simulink model "NMPC_PID"  (R2024a)
settings: Solver=FixedStepAuto  StartTime=0.0  StopTime=130  FixedStep=0.05  RelTol=1e-3
PostLoadFcn:
  | on_model_load
InitFcn:
  | on_model_start
StopFcn:
  | on_simulation_done
model workspace (MAT data in the model file):
  ActiveExperiment.Id = '85ae8ae8-3421-447e-86e6-f1860a57dbe5'
  ActiveExperiment.Name = "Two steps high noise"
  ActiveExperiment.Description = ""
  ActiveExperiment.ConstHorizonReference = 0
  ActiveExperiment.ComponentType = "scenario"
  ActiveExperiment.SimulationTime = 60
  ActiveExperiment.Subcomponents = "Disturbance"
  ActiveExperiment.Disturbance.Id = 'ccaeaedb-34fb-4469-93e3-0e771cb356d7'
  ActiveExperiment.Disturbance.Name = 'New Disturbance'
  ActiveExperiment.Disturbance.Description = ''
  ActiveExperiment.Disturbance.LibVersionHash = ''
  ActiveExperiment.Disturbance.Lib = 'csbenchlab'
  ActiveExperiment.Disturbance.LibVersion = '0.0.1'
  ActiveExperiment.Disturbance.PluginType = 'dist'
  ActiveExperiment.Disturbance.PluginName = 'Gauss'
  ActiveExperiment.Disturbance.PluginImplementation = 'mat'
  ActiveExperiment.Disturbance.ParentComponentId = '85ae8ae8-3421-447e-86e6-f1860a57dbe5'
  ActiveExperiment.Disturbance.ParentComponentType = 'scenario'
  ActiveExperiment.Disturbance.ComponentType = 'disturbance'
  ActiveExperiment.Disturbance.ParentComponentName = 'Two steps high noise'
  ActiveExperiment.SystemIc = [0; 0; 0; 0; 0; 0; 0; 0; 0; 0; 0; 0]
  ActiveExperiment.SystemParameterOverrides.payload_mass.timeseries__ = 1
  ActiveExperiment.SystemParameterOverrides.payload_mass.data = [0  0; 30  20]
  ActiveExperiment.SystemParameterOverrides.payload_location.timeseries__ = 1
  ActiveExperiment.SystemParameterOverrides.payload_location.data = [0 0 -0.15 0]
  ActiveExperiment.SystemParameterOverrides.current_speed = 0.2
  ActiveExperiment.SystemParameterOverrides.current_direction = 0.1
  ActiveExperiment.Reference = '/home/luka/fer/csbenchlab_gym/envs/marine_otter_full/data/references/85ae8ae8-3421-447e-86e6-f1860a57dbe5_ref.mat'
  ActiveExperiment.DisturbanceParameterOverrides = struct()
  ActiveExperiment.NumEvaluations = 1
  ActiveExperiment.RandomSeed = 42
  ActiveExperiment.SystemParams.payload_mass = timeseries
  ActiveExperiment.SystemParams.payload_mass.Name = 'unnamed'
  ActiveExperiment.SystemParams.payload_mass.DataInfo = tsdata.datametadata
  ActiveExperiment.SystemParams.payload_mass.DataInfo.Interpolation = tsdata.interpolation
  ActiveExperiment.SystemParams.payload_mass.DataInfo.Interpolation.Fhandle : function handle (value not decoded)
  ActiveExperiment.SystemParams.payload_mass.DataInfo.Interpolation.Name = 'linear'
  ActiveExperiment.SystemParams.payload_mass.TimeInfo = tsdata.timemetadata
  ActiveExperiment.SystemParams.payload_mass.TimeInfo.Length = 2
  ActiveExperiment.SystemParams.payload_mass.TimeInfo.DuplicateTimes = 0
  ActiveExperiment.SystemParams.payload_mass.TimeInfo.Time_ = [0; 30]
  ActiveExperiment.SystemParams.payload_mass.TimeInfo.Initialized = 1
  ActiveExperiment.SystemParams.payload_mass.QualityInfo = tsdata.qualmetadata
  ActiveExperiment.SystemParams.payload_mass.Data_ = [0; 20]
  ActiveExperiment.SystemParams.payload_location = timeseries
  ActiveExperiment.SystemParams.payload_location.Name = 'unnamed'
  ActiveExperiment.SystemParams.payload_location.DataInfo = tsdata.datametadata
  ActiveExperiment.SystemParams.payload_location.DataInfo.Interpolation = tsdata.interpolation
  ActiveExperiment.SystemParams.payload_location.DataInfo.Interpolation.Fhandle : function handle (value not decoded)
  ActiveExperiment.SystemParams.payload_location.DataInfo.Interpolation.Name = 'linear'
  ActiveExperiment.SystemParams.payload_location.TimeInfo = tsdata.timemetadata
  ActiveExperiment.SystemParams.payload_location.TimeInfo.Length = 1
  ActiveExperiment.SystemParams.payload_location.TimeInfo.DuplicateTimes = 0
  ActiveExperiment.SystemParams.payload_location.TimeInfo.Time_ = 0
  ActiveExperiment.SystemParams.payload_location.TimeInfo.Initialized = 1
  ActiveExperiment.SystemParams.payload_location.QualityInfo = tsdata.qualmetadata
  ActiveExperiment.SystemParams.payload_location.Data_ = [0 -0.15 0]
  ActiveExperiment.SystemParams.current_speed = timeseries
  ActiveExperiment.SystemParams.current_speed.Name = 'unnamed'
  ActiveExperiment.SystemParams.current_speed.DataInfo = tsdata.datametadata
  ActiveExperiment.SystemParams.current_speed.DataInfo.Interpolation = tsdata.interpolation
  ActiveExperiment.SystemParams.current_speed.DataInfo.Interpolation.Fhandle : function handle (value not decoded)
  ActiveExperiment.SystemParams.current_speed.DataInfo.Interpolation.Name = 'linear'
  ActiveExperiment.SystemParams.current_speed.TimeInfo = tsdata.timemetadata
  ActiveExperiment.SystemParams.current_speed.TimeInfo.Length = 1
  ActiveExperiment.SystemParams.current_speed.TimeInfo.DuplicateTimes = 0
  ActiveExperiment.SystemParams.current_speed.TimeInfo.Time_ = 0
  ActiveExperiment.SystemParams.current_speed.TimeInfo.Initialized = 1
  ActiveExperiment.SystemParams.current_speed.QualityInfo = tsdata.qualmetadata
  ActiveExperiment.SystemParams.current_speed.Data_ = 0.2
  ActiveExperiment.SystemParams.current_direction = timeseries
  ActiveExperiment.SystemParams.current_direction.Name = 'unnamed'
  ActiveExperiment.SystemParams.current_direction.DataInfo = tsdata.datametadata
  ActiveExperiment.SystemParams.current_direction.DataInfo.Interpolation = tsdata.interpolation
  ActiveExperiment.SystemParams.current_direction.DataInfo.Interpolation.Fhandle : function handle (value not decoded)
  ActiveExperiment.SystemParams.current_direction.DataInfo.Interpolation.Name = 'linear'
  ActiveExperiment.SystemParams.current_direction.TimeInfo = tsdata.timemetadata
  ActiveExperiment.SystemParams.current_direction.TimeInfo.Length = 1
  ActiveExperiment.SystemParams.current_direction.TimeInfo.DuplicateTimes = 0
  ActiveExperiment.SystemParams.current_direction.TimeInfo.Time_ = 0
  ActiveExperiment.SystemParams.current_direction.TimeInfo.Initialized = 1
  ActiveExperiment.SystemParams.current_direction.QualityInfo = tsdata.qualmetadata
  ActiveExperiment.SystemParams.current_direction.Data_ = 0.1
  ActiveExperiment.SystemParams.out_gain = timeseries
  ActiveExperiment.SystemParams.out_gain.Name = 'unnamed'
  ActiveExperiment.SystemParams.out_gain.DataInfo = tsdata.datametadata
  ActiveExperiment.SystemParams.out_gain.DataInfo.Interpolation = tsdata.interpolation
  ActiveExperiment.SystemParams.out_gain.DataInfo.Interpolation.Fhandle : function handle (value not decoded)
  ActiveExperiment.SystemParams.out_gain.DataInfo.Interpolation.Name = 'linear'
  ActiveExperiment.SystemParams.out_gain.TimeInfo = tsdata.timemetadata
  ActiveExperiment.SystemParams.out_gain.TimeInfo.Length = 1
  ActiveExperiment.SystemParams.out_gain.TimeInfo.DuplicateTimes = 0
  ActiveExperiment.SystemParams.out_gain.TimeInfo.Time_ = 0
  ActiveExperiment.SystemParams.out_gain.TimeInfo.Initialized = 1
  ActiveExperiment.SystemParams.out_gain.QualityInfo = tsdata.qualmetadata
  ActiveExperiment.SystemParams.out_gain.Data_ = 1
  Experiments(1).Id = '1e1e735a-ca72-47f3-9e23-ef054322de06'
  Experiments(1).Name = "Five steps perturbed high noise"
  Experiments(1).Description = ""
  Experiments(1).ConstHorizonReference = 0
  Experiments(1).ComponentType = "scenario"
  Experiments(1).SimulationTime = 60
  Experiments(1).Subcomponents = "Disturbance"
  Experiments(1).Disturbance.Id = 'd00b25fa-299c-4dde-a026-233da86bc131'
  Experiments(1).Disturbance.Name = ''
  Experiments(1).Disturbance.Description = ''
  Experiments(1).Disturbance.LibVersionHash = ''
  Experiments(1).Disturbance.Lib = 'csbenchlab'
  Experiments(1).Disturbance.LibVersion = '0.0.1'
  Experiments(1).Disturbance.PluginType = 'dist'
  Experiments(1).Disturbance.PluginName = 'Gauss'
  Experiments(1).Disturbance.PluginImplementation = 'mat'
  Experiments(1).Disturbance.ParentComponentId = '1e1e735a-ca72-47f3-9e23-ef054322de06'
  Experiments(1).Disturbance.ParentComponentName = 'Five steps perturbed high noise'
  Experiments(1).Disturbance.ParentComponentType = 'scenario'
  Experiments(1).Disturbance.ComponentType = 'disturbance'
  Experiments(1).Disturbance.DestinationPath = 'disturbances'
  Experiments(1).SystemIc = [0; 0; 0; 0; 0; 0; 0; 0; 0; 0; 0; 0]
  Experiments(1).SystemParameterOverrides.payload_mass.timeseries__ = 1
  Experiments(1).SystemParameterOverrides.payload_mass.data = [0  35; 27  35]
  Experiments(1).Reference = '/home/luka/fer/csbenchlab_gym/envs/marine_otter_full/data/references/1e1e735a-ca72-47f3-9e23-ef054322de06_ref.mat'
  Experiments(1).DisturbanceParameterOverrides = struct()
  Experiments(1).NumEvaluations = 1000
  Experiments(1).RandomSeed = 42
  Experiments(2).Id = '1e727098-795b-40af-9168-30502f01196e'
  Experiments(2).Name = "Two steps"
  Experiments(2).Description = ""
  Experiments(2).ConstHorizonReference = 0
  Experiments(2).ComponentType = "scenario"
  Experiments(2).SimulationTime = 60
  Experiments(2).Subcomponents = "Disturbance"
  Experiments(2).Disturbance = struct()
  Experiments(2).SystemIc = [0; 0; 0; 0; 0; 0; 0; 0; 0; 0; 0; 0]
  Experiments(2).SystemParameterOverrides.payload_mass.timeseries__ = 1
  Experiments(2).SystemParameterOverrides.payload_mass.data = [0  0; 27  0]
  Experiments(2).Reference = '/home/luka/fer/csbenchlab_gym/envs/marine_otter_full/data/references/1e727098-795b-40af-9168-30502f01196e_ref.mat'
  Experiments(2).DisturbanceParameterOverrides = struct()
  Experiments(2).NumEvaluations = 1
  Experiments(2).RandomSeed = 42
  Experiments(3).Id = '832a0fb6-0823-4b09-93b7-a1f8c841e784'
  Experiments(3).Name = "Sinuses"
  Experiments(3).Description = ""
  Experiments(3).ConstHorizonReference = 0
  Experiments(3).ComponentType = "scenario"
  Experiments(3).SimulationTime = 60
  Experiments(3).Subcomponents = "Disturbance"
  Experiments(3).Disturbance.Id = '6582568e-6a07-4ca1-973d-ce726013b9e5'
  Experiments(3).Disturbance.Name = ''
  Experiments(3).Disturbance.Description = ''
  Experiments(3).Disturbance.LibVersionHash = ''
  Experiments(3).Disturbance.Lib = 'csbenchlab'
  Experiments(3).Disturbance.LibVersion = '0.0.1'
  Experiments(3).Disturbance.PluginType = 'dist'
  Experiments(3).Disturbance.PluginName = 'Gauss'
  Experiments(3).Disturbance.PluginImplementation = 'mat'
  Experiments(3).Disturbance.ParentComponentId = '832a0fb6-0823-4b09-93b7-a1f8c841e784'
  Experiments(3).Disturbance.ParentComponentName = 'Sinuses'
  Experiments(3).Disturbance.ParentComponentType = 'scenario'
  Experiments(3).Disturbance.ComponentType = 'disturbance'
  Experiments(3).Disturbance.DestinationPath = 'disturbances'
  Experiments(3).SystemIc = [0; 0; 0; 0; 0; 0; 0; 0; 0; 0; 0; 0]
  Experiments(3).SystemParameterOverrides.payload_mass.timeseries__ = 1
  Experiments(3).SystemParameterOverrides.payload_mass.data = [0  35; 12  35]
  Experiments(3).Reference = '/home/luka/fer/csbenchlab_gym/envs/marine_otter_full/data/references/832a0fb6-0823-4b09-93b7-a1f8c841e784_ref.mat'
  Experiments(3).DisturbanceParameterOverrides = struct()
  Experiments(3).NumEvaluations = 1000
  Experiments(3).RandomSeed = 42
  Experiments(4).Id = '85ae8ae8-3421-447e-86e6-f1860a57dbe5'
  Experiments(4).Name = "Two steps high noise"
  Experiments(4).Description = ""
  Experiments(4).ConstHorizonReference = 0
  Experiments(4).ComponentType = "scenario"
  Experiments(4).SimulationTime = 60
  Experiments(4).Subcomponents = "Disturbance"
  Experiments(4).Disturbance.Id = 'ccaeaedb-34fb-4469-93e3-0e771cb356d7'
  Experiments(4).Disturbance.Name = 'New Disturbance'
  Experiments(4).Disturbance.Description = ''
  Experiments(4).Disturbance.LibVersionHash = ''
  Experiments(4).Disturbance.Lib = 'csbenchlab'
  Experiments(4).Disturbance.LibVersion = '0.0.1'
  Experiments(4).Disturbance.PluginType = 'dist'
  Experiments(4).Disturbance.PluginName = 'Gauss'
  Experiments(4).Disturbance.PluginImplementation = 'mat'
  Experiments(4).Disturbance.ParentComponentId = '85ae8ae8-3421-447e-86e6-f1860a57dbe5'
  Experiments(4).Disturbance.ParentComponentType = 'scenario'
  Experiments(4).Disturbance.ComponentType = 'disturbance'
  Experiments(4).Disturbance.ParentComponentName = 'Two steps high noise'
  Experiments(4).SystemIc = [0; 0; 0; 0; 0; 0; 0; 0; 0; 0; 0; 0]
  Experiments(4).SystemParameterOverrides.payload_mass.timeseries__ = 1
  Experiments(4).SystemParameterOverrides.payload_mass.data = [0  0; 30  20]
  Experiments(4).SystemParameterOverrides.payload_location.timeseries__ = 1
  Experiments(4).SystemParameterOverrides.payload_location.data = [0 0 -0.15 0]
  Experiments(4).SystemParameterOverrides.current_speed = 0.2
  Experiments(4).SystemParameterOverrides.current_direction = 0.1
  Experiments(4).Reference = '/home/luka/fer/csbenchlab_gym/envs/marine_otter_full/data/references/85ae8ae8-3421-447e-86e6-f1860a57dbe5_ref.mat'
  Experiments(4).DisturbanceParameterOverrides = struct()
  Experiments(4).NumEvaluations = 1
  Experiments(4).RandomSeed = 42
  Experiments(5).Id = '9caafca7-6b3d-4fd5-b43b-2d0badebda60'
  Experiments(5).Name = "Five steps perturbed"
  Experiments(5).Description = ""
  Experiments(5).ConstHorizonReference = 0
  Experiments(5).ComponentType = "scenario"
  Experiments(5).SimulationTime = 60
  Experiments(5).Subcomponents = "Disturbance"
  Experiments(5).Disturbance.Id = '941af73e-12e7-42cf-853d-f79bb40068e7'
  Experiments(5).Disturbance.Name = ''
  Experiments(5).Disturbance.Description = ''
  Experiments(5).Disturbance.LibVersionHash = ''
  Experiments(5).Disturbance.Lib = 'csbenchlab'
  Experiments(5).Disturbance.LibVersion = '0.0.1'
  Experiments(5).Disturbance.PluginType = 'dist'
  Experiments(5).Disturbance.PluginName = 'Gauss'
  Experiments(5).Disturbance.PluginImplementation = 'mat'
  Experiments(5).Disturbance.ParentComponentId = '9caafca7-6b3d-4fd5-b43b-2d0badebda60'
  Experiments(5).Disturbance.ParentComponentName = 'Five steps perturbed'
  Experiments(5).Disturbance.ParentComponentType = 'scenario'
  Experiments(5).Disturbance.ComponentType = 'disturbance'
  Experiments(5).Disturbance.DestinationPath = 'disturbances'
  Experiments(5).SystemIc = [0; 0; 0; 0; 0; 0; 0; 0; 0; 0; 0; 0]
  Experiments(5).SystemParameterOverrides.payload_mass.timeseries__ = 1
  Experiments(5).SystemParameterOverrides.payload_mass.data = [0  0; 27  0]
  Experiments(5).Reference = '/home/luka/fer/csbenchlab_gym/envs/marine_otter_full/data/references/9caafca7-6b3d-4fd5-b43b-2d0badebda60_ref.mat'
  Experiments(5).DisturbanceParameterOverrides = struct()
  Experiments(5).NumEvaluations = 1000
  Experiments(5).RandomSeed = 42
  Experiments(6).Id = 'd997722b-b22e-4a88-a68f-d421073cfd81'
  Experiments(6).Name = "Sinuses high noise"
  Experiments(6).Description = ""
  Experiments(6).ConstHorizonReference = 0
  Experiments(6).ComponentType = "scenario"
  Experiments(6).SimulationTime = 60
  Experiments(6).Subcomponents = "Disturbance"
  Experiments(6).Disturbance.Id = 'e3fab669-38a8-480e-9185-300544970487'
  Experiments(6).Disturbance.Name = ''
  Experiments(6).Disturbance.Description = ''
  Experiments(6).Disturbance.LibVersionHash = ''
  Experiments(6).Disturbance.Lib = 'csbenchlab'
  Experiments(6).Disturbance.LibVersion = '0.0.1'
  Experiments(6).Disturbance.PluginType = 'dist'
  Experiments(6).Disturbance.PluginName = 'Gauss'
  Experiments(6).Disturbance.PluginImplementation = 'mat'
  Experiments(6).Disturbance.ParentComponentId = 'd997722b-b22e-4a88-a68f-d421073cfd81'
  Experiments(6).Disturbance.ParentComponentName = 'Sinuses high noise'
  Experiments(6).Disturbance.ParentComponentType = 'scenario'
  Experiments(6).Disturbance.ComponentType = 'disturbance'
  Experiments(6).Disturbance.DestinationPath = 'disturbances'
  Experiments(6).SystemIc = [0; 0; 0; 0; 0; 0; 0; 0; 0; 0; 0; 0]
  Experiments(6).SystemParameterOverrides.payload_mass.timeseries__ = 1
  Experiments(6).SystemParameterOverrides.payload_mass.data = [0  35; 12  35]
  Experiments(6).Reference = '/home/luka/fer/csbenchlab_gym/envs/marine_otter_full/data/references/d997722b-b22e-4a88-a68f-d421073cfd81_ref.mat'
  Experiments(6).DisturbanceParameterOverrides = struct()
  Experiments(6).NumEvaluations = 1000
  Experiments(6).RandomSeed = 42
  GlobalReference = 0
  callbacks = dictionary
  callbacks.data.Version = 1
  callbacks.data.IsKeyCombined = 1
  callbacks.data.IsValueCombined = 1
  callbacks.data.Key = ["on_start:31b52d05-ccc9-4eab-bb0e-3c80b4e6f477"; "on_start:f41ef9e4-ba34-416c-84b6-7794956a3c04"; "on_start:9c40ba40-a30c-4d47-b6ea-332d53085db4"; "on_start:a6a9c6d3-ff58-4f5d-b7b7-6a5809d04cef"; "on_start:59d3b695-31bd-4d38-a8d0-9c2b61ca3ebd"; "on_start:68187f7d-81f5-4756-96be-de0d65363a63"; "on_start:17c1b7c7-d1b2-4e6c-bab6-21ffb9ee4dcb"; "on_start:a5c8738f-8d38-4797-a21a-203fc6d46076"; "on_load:4a0d1010-4549-4d51-b3a5-602e7c932b45"; "on_start:4a0d1010-4549-4d51-b3a5-602e7c932b45"; "on_end:4a0d1010-4549-4d51-b3a5-602e7c932b45"]
  callbacks.data.Value{1}.external_function__ = 1
  callbacks.data.Value{1}.function = 'configure_controller_params'
  callbacks.data.Value{1}.backend = 'm'
  callbacks.data.Value{1}.kwargs = struct()
  callbacks.data.Value{2}.external_function__ = 1
  callbacks.data.Value{2}.function = 'configure_controller_params'
  callbacks.data.Value{2}.backend = 'm'
  callbacks.data.Value{2}.kwargs = struct()
  callbacks.data.Value{3}.external_function__ = 1
  callbacks.data.Value{3}.function = 'configure_controller_params'
  callbacks.data.Value{3}.backend = 'm'
  callbacks.data.Value{3}.kwargs = struct()
  callbacks.data.Value{4}.external_function__ = 1
  callbacks.data.Value{4}.function = 'configure_controller_params'
  callbacks.data.Value{4}.backend = 'm'
  callbacks.data.Value{4}.kwargs = struct()
  callbacks.data.Value{5}.external_function__ = 1
  callbacks.data.Value{5}.function = 'configure_controller_params'
  callbacks.data.Value{5}.backend = 'm'
  callbacks.data.Value{5}.kwargs = struct()
  callbacks.data.Value{6}.external_function__ = 1
  callbacks.data.Value{6}.function = 'configure_controller_params'
  callbacks.data.Value{6}.backend = 'm'
  callbacks.data.Value{6}.kwargs = struct()
  callbacks.data.Value{7}.external_function__ = 1
  callbacks.data.Value{7}.function = 'configure_controller_params'
  callbacks.data.Value{7}.backend = 'm'
  callbacks.data.Value{7}.kwargs = struct()
  callbacks.data.Value{8}.external_function__ = 1
  callbacks.data.Value{8}.function = 'configure_controller_params'
  callbacks.data.Value{8}.backend = 'm'
  callbacks.data.Value{8}.kwargs = struct()
  callbacks.data.Value{9} = py.function
  callbacks.data.Value{10} = py.function
  callbacks.data.Value{11} = py.function
  env_name = 'NMPC_PID'
  extrinsic = 1
  gen_blocks.systems.systems.Name = 'CS System'
  gen_blocks.systems.systems.Handle = 'NMPC_PID/CS System'
  gen_blocks.systems.systems.Path = 'NMPC_PID/CS System'
  gen_blocks.systems.systems.Disturbance = []
  gen_blocks.systems.systems.Id = "4a0d1010-4549-4d51-b3a5-602e7c932b45"
  gen_blocks.systems.systems.Components.Name = 'Otter'
  gen_blocks.systems.systems.Components.Handle = 1179.08288574
  gen_blocks.systems.systems.Components.Path = 'NMPC_PID/CS System/Otter'
  gen_blocks.systems.systems.Components.Id = "4a0d1010-4549-4d51-b3a5-602e7c932b45"
  gen_blocks.systems.systems.Components.LibPath = "marine_lib_sys/Otter"
  gen_blocks.systems.systems.SignalSubsystem = []
  gen_blocks.systems.dims.Inputs = 2
  gen_blocks.systems.dims.Outputs = 12
  gen_blocks.controllers.Name = 'CS Controller'
  gen_blocks.controllers.Handle = 'NMPC_PID/CS Controller'
  gen_blocks.controllers.Path = 'NMPC_PID/CS Controller'
  gen_blocks.controllers.Id = "8582e3e1-de85-466e-b412-44a269ccd2bf"
  gen_blocks.controllers.Components.Name = 'PID'
  gen_blocks.controllers.Components.Handle = 7921.01660156
  gen_blocks.controllers.Components.Path = 'NMPC_PID/CS Controller/PID'
  gen_blocks.controllers.Components.Id = "8582e3e1-de85-466e-b412-44a269ccd2bf"
  gen_blocks.controllers.Components.LibPath = "csbenchlab_ctl/PID"
  gen_blocks.controllers.Components.RefExtractor.Path = 'NMPC_PID/CS Controller/ref_extractor_1'
  gen_blocks.controllers.IoHandles.inport_y.h = 1033.08984375
  gen_blocks.controllers.IoHandles.inport_y.p.Inport = []
  gen_blocks.controllers.IoHandles.inport_y.p.Outport = 1034.08666992
  gen_blocks.controllers.IoHandles.inport_y.p.Enable = []
  gen_blocks.controllers.IoHandles.inport_y.p.Trigger = []
  gen_blocks.controllers.IoHandles.inport_y.p.State = []
  gen_blocks.controllers.IoHandles.inport_y.p.LConn = []
  gen_blocks.controllers.IoHandles.inport_y.p.RConn = []
  gen_blocks.controllers.IoHandles.inport_y.p.Ifaction = []
  gen_blocks.controllers.IoHandles.inport_y.p.Reset = []
  gen_blocks.controllers.IoHandles.inport_y.p.Event = []
  gen_blocks.controllers.IoHandles.inport_yref.h = 1031.09008789
  gen_blocks.controllers.IoHandles.inport_yref.p.Inport = []
  gen_blocks.controllers.IoHandles.inport_yref.p.Outport = 1032.08898926
  gen_blocks.controllers.IoHandles.inport_yref.p.Enable = []
  gen_blocks.controllers.IoHandles.inport_yref.p.Trigger = []
  gen_blocks.controllers.IoHandles.inport_yref.p.State = []
  gen_blocks.controllers.IoHandles.inport_yref.p.LConn = []
  gen_blocks.controllers.IoHandles.inport_yref.p.RConn = []
  gen_blocks.controllers.IoHandles.inport_yref.p.Ifaction = []
  gen_blocks.controllers.IoHandles.inport_yref.p.Reset = []
  gen_blocks.controllers.IoHandles.inport_yref.p.Event = []
  gen_blocks.controllers.IoHandles.outport_u.h = 1035.08679199
  gen_blocks.controllers.IoHandles.outport_u.p.Inport = 1036.08850098
  gen_blocks.controllers.IoHandles.outport_u.p.Outport = []
  gen_blocks.controllers.IoHandles.outport_u.p.Enable = []
  gen_blocks.controllers.IoHandles.outport_u.p.Trigger = []
  gen_blocks.controllers.IoHandles.outport_u.p.State = []
  gen_blocks.controllers.IoHandles.outport_u.p.LConn = []
  gen_blocks.controllers.IoHandles.outport_u.p.RConn = []
  gen_blocks.controllers.IoHandles.outport_u.p.Ifaction = []
  gen_blocks.controllers.IoHandles.outport_u.p.Reset = []
  gen_blocks.controllers.IoHandles.outport_u.p.Event = []
  gen_blocks.controllers.IoHandles.outport_log.h = 1037.08850098
  gen_blocks.controllers.IoHandles.outport_log.p.Inport = 1038.08740234
  gen_blocks.controllers.IoHandles.outport_log.p.Outport = []
  gen_blocks.controllers.IoHandles.outport_log.p.Enable = []
  gen_blocks.controllers.IoHandles.outport_log.p.Trigger = []
  gen_blocks.controllers.IoHandles.outport_log.p.State = []
  gen_blocks.controllers.IoHandles.outport_log.p.LConn = []
  gen_blocks.controllers.IoHandles.outport_log.p.RConn = []
  gen_blocks.controllers.IoHandles.outport_log.p.Ifaction = []
  gen_blocks.controllers.IoHandles.outport_log.p.Reset = []
  gen_blocks.controllers.IoHandles.outport_log.p.Event = []
  gen_blocks.controllers.IoHandles.in_demux.p.Inport = 1436.0949707
  gen_blocks.controllers.IoHandles.in_demux.p.Outport = [1437.0904541 1438.09033203 1449.0925293 1450.09375 1451.09008789 1452.09130859 1453.08947754 1454.09729004 1455.09594727 1456.09484863 1457.09289551 1458.09545898]
  gen_blocks.controllers.IoHandles.in_demux.p.Enable = []
  gen_blocks.controllers.IoHandles.in_demux.p.Trigger = []
  gen_blocks.controllers.IoHandles.in_demux.p.State = []
  gen_blocks.controllers.IoHandles.in_demux.p.LConn = []
  gen_blocks.controllers.IoHandles.in_demux.p.RConn = []
  gen_blocks.controllers.IoHandles.in_demux.p.Ifaction = []
  gen_blocks.controllers.IoHandles.in_demux.p.Reset = []
  gen_blocks.controllers.IoHandles.in_demux.p.Event = []
  gen_blocks.controllers.IoHandles.in_demux.h = 1435.09838867
  gen_blocks.controllers.IoHandles.in_demux_ref.p.Inport = 1432.09680176
  gen_blocks.controllers.IoHandles.in_demux_ref.p.Outport = [1433.09960938 1434.10009766 1439.0904541 1440.09106445 1441.09228516 1442.09130859 1443.09155273 1444.09118652 1445.0925293 1446.09729004 1447.09594727 1448.09460449]
  gen_blocks.controllers.IoHandles.in_demux_ref.p.Enable = []
  gen_blocks.controllers.IoHandles.in_demux_ref.p.Trigger = []
  gen_blocks.controllers.IoHandles.in_demux_ref.p.State = []
  gen_blocks.controllers.IoHandles.in_demux_ref.p.LConn = []
  gen_blocks.controllers.IoHandles.in_demux_ref.p.RConn = []
  gen_blocks.controllers.IoHandles.in_demux_ref.p.Ifaction = []
  gen_blocks.controllers.IoHandles.in_demux_ref.p.Reset = []
  gen_blocks.controllers.IoHandles.in_demux_ref.p.Event = []
  gen_blocks.controllers.IoHandles.in_demux_ref.h = 1431.0949707
  gen_blocks.controllers.IoHandles.out_mux.p.Inport = [1463.09765625 1465.09057617]
  gen_blocks.controllers.IoHandles.out_mux.p.Outport = 1466.09521484
  gen_blocks.controllers.IoHandles.out_mux.p.Enable = []
  gen_blocks.controllers.IoHandles.out_mux.p.Trigger = []
  gen_blocks.controllers.IoHandles.out_mux.p.State = []
  gen_blocks.controllers.IoHandles.out_mux.p.LConn = []
  gen_blocks.controllers.IoHandles.out_mux.p.RConn = []
  gen_blocks.controllers.IoHandles.out_mux.p.Ifaction = []
  gen_blocks.controllers.IoHandles.out_mux.p.Reset = []
  gen_blocks.controllers.IoHandles.out_mux.p.Event = []
  gen_blocks.controllers.IoHandles.out_mux.h = 1462.09448242
  gen_blocks.controllers.IoHandles.out_mux_log.p.Inport = 1471.09155273
  gen_blocks.controllers.IoHandles.out_mux_log.p.Outport = 7511.01745605
  gen_blocks.controllers.IoHandles.out_mux_log.p.Enable = []
  gen_blocks.controllers.IoHandles.out_mux_log.p.Trigger = []
  gen_blocks.controllers.IoHandles.out_mux_log.p.State = []
  gen_blocks.controllers.IoHandles.out_mux_log.p.LConn = []
  gen_blocks.controllers.IoHandles.out_mux_log.p.RConn = []
  gen_blocks.controllers.IoHandles.out_mux_log.p.Ifaction = []
  gen_blocks.controllers.IoHandles.out_mux_log.p.Reset = []
  gen_blocks.controllers.IoHandles.out_mux_log.p.Event = []
  gen_blocks.controllers.IoHandles.out_mux_log.h = 1470.08764648
  gen_blocks.controllers.IoHandles.ref_extractors.h = 9020.01672363
  gen_blocks.controllers.IoHandles.ref_extractors.name = 'ref_extractor_1'
  gen_blocks.controllers.IoHandles.ref_extractors.p.Inport = 9023.01660156
  gen_blocks.controllers.IoHandles.ref_extractors.p.Outport = 9149.01818848
  gen_blocks.controllers.IoHandles.ref_extractors.p.Enable = []
  gen_blocks.controllers.IoHandles.ref_extractors.p.Trigger = []
  gen_blocks.controllers.IoHandles.ref_extractors.p.State = []
  gen_blocks.controllers.IoHandles.ref_extractors.p.LConn = []
  gen_blocks.controllers.IoHandles.ref_extractors.p.RConn = []
  gen_blocks.controllers.IoHandles.ref_extractors.p.Ifaction = []
  gen_blocks.controllers.IoHandles.ref_extractors.p.Reset = []
  gen_blocks.controllers.IoHandles.ref_extractors.p.Event = []
  gen_blocks.controllers.IoHandles.adapters.in_mux.h = 9208.01599121
  gen_blocks.controllers.IoHandles.adapters.in_mux.p.Inport = [9210.01586914 9211.01696777]
  gen_blocks.controllers.IoHandles.adapters.in_mux.p.Outport = 9212.0168457
  gen_blocks.controllers.IoHandles.adapters.in_mux.p.Enable = []
  gen_blocks.controllers.IoHandles.adapters.in_mux.p.Trigger = []
  gen_blocks.controllers.IoHandles.adapters.in_mux.p.State = []
  gen_blocks.controllers.IoHandles.adapters.in_mux.p.LConn = []
  gen_blocks.controllers.IoHandles.adapters.in_mux.p.RConn = []
  gen_blocks.controllers.IoHandles.adapters.in_mux.p.Ifaction = []
  gen_blocks.controllers.IoHandles.adapters.in_mux.p.Reset = []
  gen_blocks.controllers.IoHandles.adapters.in_mux.p.Event = []
  gen_blocks.controllers.IoHandles.adapters.in_mux_ref.h = 9213.01550293
  gen_blocks.controllers.IoHandles.adapters.in_mux_ref.p.Inport = [9214.01623535 9215.01696777]
  gen_blocks.controllers.IoHandles.adapters.in_mux_ref.p.Outport = 10245.0172119
  gen_blocks.controllers.IoHandles.adapters.in_mux_ref.p.Enable = []
  gen_blocks.controllers.IoHandles.adapters.in_mux_ref.p.Trigger = []
  gen_blocks.controllers.IoHandles.adapters.in_mux_ref.p.State = []
  gen_blocks.controllers.IoHandles.adapters.in_mux_ref.p.LConn = []
  gen_blocks.controllers.IoHandles.adapters.in_mux_ref.p.RConn = []
  gen_blocks.controllers.IoHandles.adapters.in_mux_ref.p.Ifaction = []
  gen_blocks.controllers.IoHandles.adapters.in_mux_ref.p.Reset = []
  gen_blocks.controllers.IoHandles.adapters.in_mux_ref.p.Event = []
  gen_blocks.controllers.IoHandles.adapters.out_demux.h = 10250.0166016
  gen_blocks.controllers.IoHandles.adapters.out_demux.p.Inport = 10368.0174561
  gen_blocks.controllers.IoHandles.adapters.out_demux.p.Outport = [10369.0168457 10370.0164795]
  gen_blocks.controllers.IoHandles.adapters.out_demux.p.Enable = []
  gen_blocks.controllers.IoHandles.adapters.out_demux.p.Trigger = []
  gen_blocks.controllers.IoHandles.adapters.out_demux.p.State = []
  gen_blocks.controllers.IoHandles.adapters.out_demux.p.LConn = []
  gen_blocks.controllers.IoHandles.adapters.out_demux.p.RConn = []
  gen_blocks.controllers.IoHandles.adapters.out_demux.p.Ifaction = []
  gen_blocks.controllers.IoHandles.adapters.out_demux.p.Reset = []
  gen_blocks.controllers.IoHandles.adapters.out_demux.p.Event = []
  gen_blocks.controllers.IoHandles.adapters.scopes.y.h = 10373.0178223
  gen_blocks.controllers.IoHandles.adapters.scopes.y.p.Inport = [10375.0168457 10380.0159912]
  gen_blocks.controllers.IoHandles.adapters.scopes.y.p.Outport = []
  gen_blocks.controllers.IoHandles.adapters.scopes.y.p.Enable = []
  gen_blocks.controllers.IoHandles.adapters.scopes.y.p.Trigger = []
  gen_blocks.controllers.IoHandles.adapters.scopes.y.p.State = []
  gen_blocks.controllers.IoHandles.adapters.scopes.y.p.LConn = []
  gen_blocks.controllers.IoHandles.adapters.scopes.y.p.RConn = []
  gen_blocks.controllers.IoHandles.adapters.scopes.y.p.Ifaction = []
  gen_blocks.controllers.IoHandles.adapters.scopes.y.p.Reset = []
  gen_blocks.controllers.IoHandles.adapters.scopes.y.p.Event = []
  gen_blocks.controllers.IoHandles.adapters.scopes.u.h = 10376.0195312
  gen_blocks.controllers.IoHandles.adapters.scopes.u.p.Inport = 10378.0200195
  gen_blocks.controllers.IoHandles.adapters.scopes.u.p.Outport = []
  gen_blocks.controllers.IoHandles.adapters.scopes.u.p.Enable = []
  gen_blocks.controllers.IoHandles.adapters.scopes.u.p.Trigger = []
  gen_blocks.controllers.IoHandles.adapters.scopes.u.p.State = []
  gen_blocks.controllers.IoHandles.adapters.scopes.u.p.LConn = []
  gen_blocks.controllers.IoHandles.adapters.scopes.u.p.RConn = []
  gen_blocks.controllers.IoHandles.adapters.scopes.u.p.Ifaction = []
  gen_blocks.controllers.IoHandles.adapters.scopes.u.p.Reset = []
  gen_blocks.controllers.IoHandles.adapters.scopes.u.p.Event = []
  gen_blocks.controllers.IoHandles.adapters.cont.h = 7921.01660156
  gen_blocks.controllers.IoHandles.adapters.cont.p.Inport = [7924.01269531 7925.01489258 7926.01501465]
  gen_blocks.controllers.IoHandles.adapters.cont.p.Outport = [9012.01733398 9013.01733398]
  gen_blocks.controllers.IoHandles.adapters.cont.p.Enable = []
  gen_blocks.controllers.IoHandles.adapters.cont.p.Trigger = []
  gen_blocks.controllers.IoHandles.adapters.cont.p.State = []
  gen_blocks.controllers.IoHandles.adapters.cont.p.LConn = []
  gen_blocks.controllers.IoHandles.adapters.cont.p.RConn = []
  gen_blocks.controllers.IoHandles.adapters.cont.p.Ifaction = []
  gen_blocks.controllers.IoHandles.adapters.cont.p.Reset = []
  gen_blocks.controllers.IoHandles.adapters.cont.p.Event = []
  gen_blocks.controllers.IoHandles.adapters.Mux.Inputs = [1 6]
  gen_blocks.controllers.IoHandles.adapters.Mux.Outputs = [1 2]
  gen_blocks.controllers.Estimator = []
  gen_blocks.controllers.Disturbance = []
  gen_blocks.controllers.SignalSubsystem = []
  gen_blocks.cs_blocks = {'NMPC_PID/CS Controller'; 'NMPC_PID/CS Controller/PID'; 'NMPC_PID/CS System'; 'NMPC_PID/CS System/Otter'}
  gen_data_dictionary = Simulink.data.Dictionary
  id_to_params_path_map = dictionary
  id_to_params_path_map.data.Version = 1
  id_to_params_path_map.data.IsKeyCombined = 1
  id_to_params_path_map.data.IsValueCombined = 1
  id_to_params_path_map.data.Key = ["4a0d1010-4549-4d51-b3a5-602e7c932b45"; "8582e3e1-de85-466e-b412-44a269ccd2bf"; "d00b25fa-299c-4dde-a026-233da86bc131"; "6582568e-6a07-4ca1-973d-ce726013b9e5"; "ccaeaedb-34fb-4469-93e3-0e771cb356d7"; "941af73e-12e7-42cf-853d-f79bb40068e7"; "e3fab669-38a8-480e-9185-300544970487"]
  id_to_params_path_map.data.Value = ["NMPC_PID_params.sys.Otter"; "NMPC_PID_params.ctl.PID"; "NMPC_PID_params.Subcomponents.FiveStepsPerturbedHighNoise.x"; "NMPC_PID_params.Subcomponents.Sinuses.x"; "NMPC_PID_params.Subcomponents.TwoStepsHighNoise.NewDisturbance"; "NMPC_PID_params.Subcomponents.FiveStepsPerturbed.x"; "NMPC_PID_params.Subcomponents.SinusesHighNoise.x"]
  model_info.Metadata.Id = "ab4d190f-a5ed-423c-bf24-5e5b13858970"
  model_info.Metadata.Name = "marine_otter_full"
  model_info.Metadata.Version = "0.1"
  model_info.Metadata.Ts = 0.05
  model_info.Metadata.ComponentType = "metadata"
  model_info.Metadata.CoderExtrinsic = 1
  model_info.Controllers.Id = "8582e3e1-de85-466e-b412-44a269ccd2bf"
  model_info.Controllers.Name = "PID"
  model_info.Controllers.Description = ""
  model_info.Controllers.LibVersionHash = ""
  model_info.Controllers.Lib = "csbenchlab"
  model_info.Controllers.LibVersion = "0.0.1"
  model_info.Controllers.PluginType = "ctl"
  model_info.Controllers.PluginName = "PID"
  model_info.Controllers.IsComposable = 0
  model_info.Controllers.RefHorizon = 0
  model_info.Controllers.Mux.Inputs = [1 6]
  model_info.Controllers.Mux.Outputs = [1 2]
  model_info.Controllers.Subcomponents = "Subcontrollers"
  model_info.Controllers.Disturbance = struct()
  model_info.Controllers.ComponentType = "controller"
  model_info.Controllers.PluginImplementation = "slx"
  model_info.Controllers.Subcontrollers = []
  model_info.System.Id = "4a0d1010-4549-4d51-b3a5-602e7c932b45"
  model_info.System.Name = "Otter"
  model_info.System.Description = ""
  model_info.System.LibVersionHash = ""
  model_info.System.Lib = "marine_lib"
  model_info.System.LibVersion = "0.0.1"
  model_info.System.PluginType = "sys"
  model_info.System.PluginName = "Otter"
  model_info.System.Subcomponents = "Disturbance"
  model_info.System.Disturbance = struct()
  model_info.System.ComponentType = "system"
  model_info.System.PluginImplementation = "slx"
  model_info.Metrics.Id = "9c8fc09b-5b47-4f25-8326-e915b50c92f8"
  model_info.Metrics.Name = "Plot out wit reference"
  model_info.Metrics.Description = ""
  model_info.Metrics.ComponentType = "metric"
  model_info.Experiments(1).Id = "1e1e735a-ca72-47f3-9e23-ef054322de06"
  model_info.Experiments(1).Name = "Five steps perturbed high noise"
  model_info.Experiments(1).Description = ""
  model_info.Experiments(1).ConstHorizonReference = 0
  model_info.Experiments(1).ComponentType = "scenario"
  model_info.Experiments(1).SimulationTime = 60
  model_info.Experiments(1).Subcomponents = "Disturbance"
  model_info.Experiments(1).Disturbance.Id = "d00b25fa-299c-4dde-a026-233da86bc131"
  model_info.Experiments(1).Disturbance.Name = ""
  model_info.Experiments(1).Disturbance.Description = ""
  model_info.Experiments(1).Disturbance.LibVersionHash = ""
  model_info.Experiments(1).Disturbance.Lib = "csbenchlab"
  model_info.Experiments(1).Disturbance.LibVersion = "0.0.1"
  model_info.Experiments(1).Disturbance.PluginType = "dist"
  model_info.Experiments(1).Disturbance.PluginName = "Gauss"
  model_info.Experiments(1).Disturbance.PluginImplementation = "mat"
  model_info.Experiments(1).Disturbance.ParentComponentId = "1e1e735a-ca72-47f3-9e23-ef054322de06"
  model_info.Experiments(1).Disturbance.ParentComponentName = "Five steps perturbed high noise"
  model_info.Experiments(1).Disturbance.ParentComponentType = "scenario"
  model_info.Experiments(1).Disturbance.ComponentType = "disturbance"
  model_info.Experiments(1).Disturbance.DestinationPath = "disturbances"
  model_info.Experiments(2).Id = "1e727098-795b-40af-9168-30502f01196e"
  model_info.Experiments(2).Name = "Two steps"
  model_info.Experiments(2).Description = ""
  model_info.Experiments(2).ConstHorizonReference = 0
  model_info.Experiments(2).ComponentType = "scenario"
  model_info.Experiments(2).SimulationTime = 60
  model_info.Experiments(2).Subcomponents = "Disturbance"
  model_info.Experiments(2).Disturbance = struct()
  model_info.Experiments(3).Id = "832a0fb6-0823-4b09-93b7-a1f8c841e784"
  model_info.Experiments(3).Name = "Sinuses"
  model_info.Experiments(3).Description = ""
  model_info.Experiments(3).ConstHorizonReference = 0
  model_info.Experiments(3).ComponentType = "scenario"
  model_info.Experiments(3).SimulationTime = 60
  model_info.Experiments(3).Subcomponents = "Disturbance"
  model_info.Experiments(3).Disturbance.Id = "6582568e-6a07-4ca1-973d-ce726013b9e5"
  model_info.Experiments(3).Disturbance.Name = ""
  model_info.Experiments(3).Disturbance.Description = ""
  model_info.Experiments(3).Disturbance.LibVersionHash = ""
  model_info.Experiments(3).Disturbance.Lib = "csbenchlab"
  model_info.Experiments(3).Disturbance.LibVersion = "0.0.1"
  model_info.Experiments(3).Disturbance.PluginType = "dist"
  model_info.Experiments(3).Disturbance.PluginName = "Gauss"
  model_info.Experiments(3).Disturbance.PluginImplementation = "mat"
  model_info.Experiments(3).Disturbance.ParentComponentId = "832a0fb6-0823-4b09-93b7-a1f8c841e784"
  model_info.Experiments(3).Disturbance.ParentComponentName = "Sinuses"
  model_info.Experiments(3).Disturbance.ParentComponentType = "scenario"
  model_info.Experiments(3).Disturbance.ComponentType = "disturbance"
  model_info.Experiments(3).Disturbance.DestinationPath = "disturbances"
  model_info.Experiments(4).Id = "85ae8ae8-3421-447e-86e6-f1860a57dbe5"
  model_info.Experiments(4).Name = "Two steps high noise"
  model_info.Experiments(4).Description = ""
  model_info.Experiments(4).ConstHorizonReference = 0
  model_info.Experiments(4).ComponentType = "scenario"
  model_info.Experiments(4).SimulationTime = 60
  model_info.Experiments(4).Subcomponents = "Disturbance"
  model_info.Experiments(4).Disturbance.Id = "ccaeaedb-34fb-4469-93e3-0e771cb356d7"
  model_info.Experiments(4).Disturbance.Name = "New Disturbance"
  model_info.Experiments(4).Disturbance.Description = ""
  model_info.Experiments(4).Disturbance.LibVersionHash = ""
  model_info.Experiments(4).Disturbance.Lib = "csbenchlab"
  model_info.Experiments(4).Disturbance.LibVersion = "0.0.1"
  model_info.Experiments(4).Disturbance.PluginType = "dist"
  model_info.Experiments(4).Disturbance.PluginName = "Gauss"
  model_info.Experiments(4).Disturbance.PluginImplementation = "mat"
  model_info.Experiments(4).Disturbance.ParentComponentId = "85ae8ae8-3421-447e-86e6-f1860a57dbe5"
  model_info.Experiments(4).Disturbance.ParentComponentType = "scenario"
  model_info.Experiments(4).Disturbance.ComponentType = "disturbance"
  model_info.Experiments(4).Disturbance.DestinationPath = "disturbances"
  model_info.Experiments(4).Disturbance.ParentComponentName = "Two steps high noise"
  model_info.Experiments(5).Id = "9caafca7-6b3d-4fd5-b43b-2d0badebda60"
  model_info.Experiments(5).Name = "Five steps perturbed"
  model_info.Experiments(5).Description = ""
  model_info.Experiments(5).ConstHorizonReference = 0
  model_info.Experiments(5).ComponentType = "scenario"
  model_info.Experiments(5).SimulationTime = 60
  model_info.Experiments(5).Subcomponents = "Disturbance"
  model_info.Experiments(5).Disturbance.Id = "941af73e-12e7-42cf-853d-f79bb40068e7"
  model_info.Experiments(5).Disturbance.Name = ""
  model_info.Experiments(5).Disturbance.Description = ""
  model_info.Experiments(5).Disturbance.LibVersionHash = ""
  model_info.Experiments(5).Disturbance.Lib = "csbenchlab"
  model_info.Experiments(5).Disturbance.LibVersion = "0.0.1"
  model_info.Experiments(5).Disturbance.PluginType = "dist"
  model_info.Experiments(5).Disturbance.PluginName = "Gauss"
  model_info.Experiments(5).Disturbance.PluginImplementation = "mat"
  model_info.Experiments(5).Disturbance.ParentComponentId = "9caafca7-6b3d-4fd5-b43b-2d0badebda60"
  model_info.Experiments(5).Disturbance.ParentComponentName = "Five steps perturbed"
  model_info.Experiments(5).Disturbance.ParentComponentType = "scenario"
  model_info.Experiments(5).Disturbance.ComponentType = "disturbance"
  model_info.Experiments(5).Disturbance.DestinationPath = "disturbances"
  model_info.Experiments(6).Id = "d997722b-b22e-4a88-a68f-d421073cfd81"
  model_info.Experiments(6).Name = "Sinuses high noise"
  model_info.Experiments(6).Description = ""
  model_info.Experiments(6).ConstHorizonReference = 0
  model_info.Experiments(6).ComponentType = "scenario"
  model_info.Experiments(6).SimulationTime = 60
  model_info.Experiments(6).Subcomponents = "Disturbance"
  model_info.Experiments(6).Disturbance.Id = "e3fab669-38a8-480e-9185-300544970487"
  model_info.Experiments(6).Disturbance.Name = ""
  model_info.Experiments(6).Disturbance.Description = ""
  model_info.Experiments(6).Disturbance.LibVersionHash = ""
  model_info.Experiments(6).Disturbance.Lib = "csbenchlab"
  model_info.Experiments(6).Disturbance.LibVersion = "0.0.1"
  model_info.Experiments(6).Disturbance.PluginType = "dist"
  model_info.Experiments(6).Disturbance.PluginName = "Gauss"
  model_info.Experiments(6).Disturbance.PluginImplementation = "mat"
  model_info.Experiments(6).Disturbance.ParentComponentId = "d997722b-b22e-4a88-a68f-d421073cfd81"
  model_info.Experiments(6).Disturbance.ParentComponentName = "Sinuses high noise"
  model_info.Experiments(6).Disturbance.ParentComponentType = "scenario"
  model_info.Experiments(6).Disturbance.ComponentType = "disturbance"
  model_info.Experiments(6).Disturbance.DestinationPath = "disturbances"
  model_info.Path = '/home/luka/fer/csbenchlab_gym/envs/marine_otter_full'
  model_info.IsControlEnvironment = 0
  model_type = 'scenario'
  old_params : object (value not decoded)
undefined symbols (not defined in the file): rpp_params
libraries: csbenchlab_ctl x1, marine_lib_sys x1, cmmi_lib x1
PostSaveFcn:
  | on_model_save
settings Model: DataDictionary=NMPC_PID_bus_types.sldd  Creator=luka  LastModifiedBy=luka

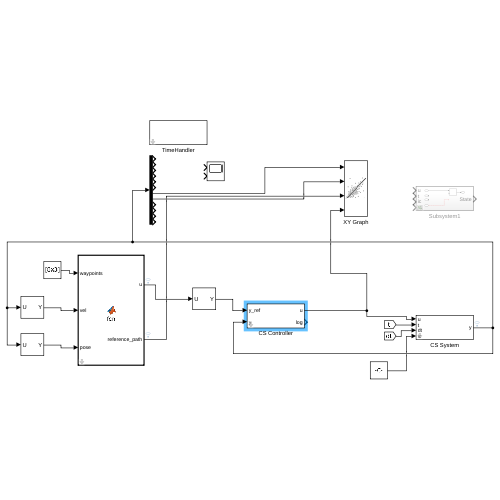
[thumbnail: Simulink's stored preview of the top-level diagram]
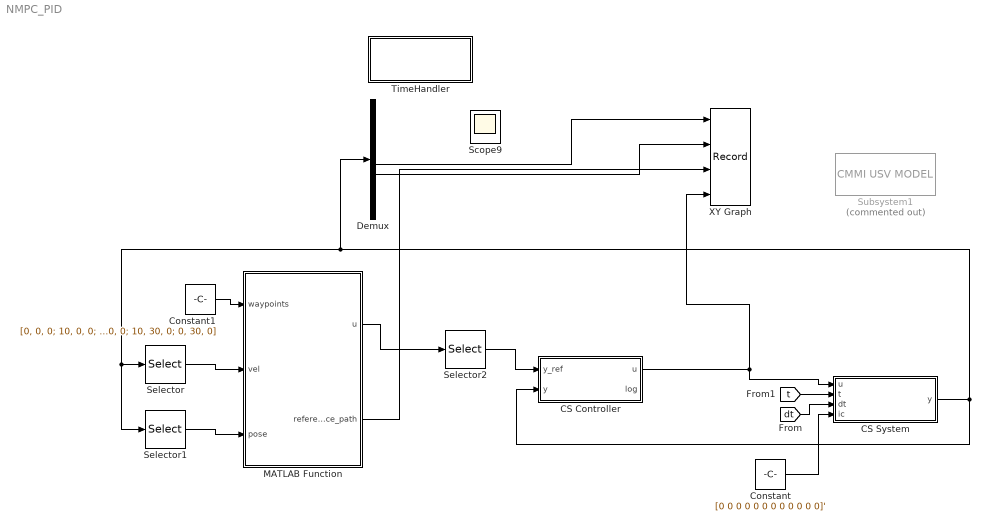
== system NMPC_PID ==
  CS Controller : Subsystem  Tag=__cs_template;__cs_comptype:ctl
      mask DialogControl ParameterGroupVar Prompt: Params
  CS System : Subsystem  Tag=__cs_template;__cs_comptype:sys
      mask DialogControl ParameterGroupVar Prompt: Params
  Constant : Constant  Value=[0 0 0 0 0 0 0 0 0 0 0 0]'
  Constant1 : Constant  Value=[0, 0, 0; 10, 0, 0; 10 10, 0; 0, 10, 0; 0, 20, 0; 10, 20, 0; 10, 30, 0; 0, 30, 0]
  Demux : Demux  Outputs=12
  MATLAB Function : MATLAB Function  TreatAsAtomicUnit=on  SystemSampleTime=0.8  mask{params=rpp_params}
  Scope9 : Scope  NumInputPorts=2
  Selector : Selector  InputPortWidth=12  IndexOptions=Index vector (dialog)  Indices=[1 2 6]  OutputSizes=1
  Selector1 : Selector  InputPortWidth=12  IndexOptions=Index vector (dialog)  Indices=[7 8 12]  OutputSizes=1
  Selector2 : Selector  NumberOfDimensions=2  InputPortWidth=12  IndexOptions=Index vector (dialog),Select all  Indices=1,1  OutputSizes=1,1
  Subsystem1 : cmmi_lib/CMMI USV MODEL  Commented=on  SystemSampleTime=-1  VariantActivationTime=update diagram  AllowFlexibleInterface=on  Latency=0  AutoFrameSizeCalculation=off
      link override Subsystem/Saturation: UpperLimit=1  LowerLimit=-1
  TimeHandler : Subsystem
      mask DialogControl ParameterGroupVar Prompt: Params
  XY Graph : Record  FileSettingsInternal="{\"entries\":[{\"content\":{\"excelSettings\":{\"content\":{},\"type\":\"Streamout.ExcelSettings\"}},\"type\":\"Streamout.FileSettingStorage\",\"uuid\":\"\"}],\"packageUris\":[\"http:\\/\\/schema.mathworks.com\\/mf0\\/streamout_blocks\\/R2020a\"],\"version\":\"1.0\"}"  Layout=[1 1]  SignalsInternal="{\"entries\":[{\"content\":{\"signals\":[{\"content\":{\"blockPath\":[],\"dimensions\":[1],\"domain\":\"\",\"lineColor\":\"#4dbeee\",\"lineWidth\":2,\"plots\":[ 1 ],\"port\":1,\"sid\":[\"\"],\"signalID\":1,\"signalName\":\"Demux:7\"},\"type\":\"RecordBlkView.Signal\",\"uuid\":\"\"},{\"content\":{\"blockPath\":[],\"dimensions\":[1],\"domain\":\"\",\"lineColor\":\"#a2142f\",\"lineWidth\":2,\"plots\":[ 1 ],\"port\":2,\"sid\":[\"\"],\"signalID\":2,\"signalName\":\"Demux:8\"},\"type\":\"RecordBlkView.Signal\",\"uuid\":\"\"},{\"content\":{\"blockPath\":[],\"dimensions\":[701,3],\"domain\":\"\",\"hasChildren\":true,\"lineColor\":\"#a2142f\",\"lineWidth\":2,\"port\":3,\"sid\":[\"\"],\"signalID\":3,\"signalName\":\"MATLAB Function:2\"},\"type\":\"RecordBlkView.Signal\",\"uuid\":\"\"},{\"content\":{\"blockPath\":[],\"channel\":[1,1],\"dimensions\":[701,3],\"domain\":\"\",\"lineColor\":\"#ff6929\",\"lineWidth\":2,\"parentID\":3,\"port\":3,\"sid\":[\"\"],\"signalID\":4,\"signalName\":\"MATLAB Function:2\"},\"type\":\"RecordBlkView.Signal\",\"uuid\":\"\"},{\"content\":{\"blockPath\":[],\"dimensions\":[2],\"domain\":\"\",\"hasChildren\":true,\"lineColor\":\"#ff6929\",\"lineWidth\":2,\"port\":4,\"sid\":[\"\"],\"signalID\":5,\"signalName\":\"CS Controller:1\"},\"type\":\"RecordBlkView.Signal\",\"uuid\":\"\"},{\"content\":{\"blockPath\":[],\"channel\":[1],\"dimensions\":[2],\"domain\":\"\",\"lineColor\":\"#64d413\",\"lineWidth\":2,\"parentID\":5,\"port\":4,\"sid\":[\"\"],\"signalID\":6,\"signalName\":\"CS Controller:1\"},\"type\":\"RecordBlkView.Signal\",\"uuid\":\"\"},{\"content\":{\"blockPath\":[],\"channel\":[2],\"dimensions\":[2],\"domain\":\"\",\"lineColor\":\"#ff13a6\",\"lineWidth\":2,\"parentID\":5,\"port\":4,\"sid\":[\"\"],\"signalID\":7,\"signalName\":\"CS Controller:1\"},\"type\":\"RecordBlkView.Signal\",\"uuid\":\"\"}]},\"type\":\"RecordBlkView.InputSignals\",\"uuid\":\"\"}],\"packageUris\":[\"http:\\/\\/schema.mathworks.com\\/mf0\\/streamout_blocks\\/R2020a\"],\"version\":\"1.0\"}"  VisualizationBindings="{\"xyplotplugin\":{\"info\":[{\"series\":[{\"bindingParametersList\":[{\"parameter\":\"X-Axis\",\"signalID\":1,\"signalName\":\"Demux:7\"},{\"parameter\":\"Y-Axis\",\"signalID\":2,\"signalName\":\"Demux:8\"}],\"seriesID\":0}],\"subplotID\":1}]}}"  CompatibilityTag=XY
  wires:
  Constant1/1 -> MATLAB Function/1(waypoints)
  Selector/1 -> MATLAB Function/2(vel)
  Selector1/1 -> MATLAB Function/3(pose)
  CS Controller/1(u) -> CS System/1(u), XY Graph/4
  [dt] -> CS System/3(dt)
  [t] -> CS System/2(t)
  Constant/1 -> CS System/4(ic)
  CS System/1(y) -> CS Controller/2(y), Selector1/1, Selector/1, Demux/1
  MATLAB Function/2(reference_path) -> XY Graph/3
  Demux/7 -> XY Graph/1
  Demux/8 -> XY Graph/2
  MATLAB Function/1(u) -> Selector2/1
  Selector2/1 -> CS Controller/1(y_ref)

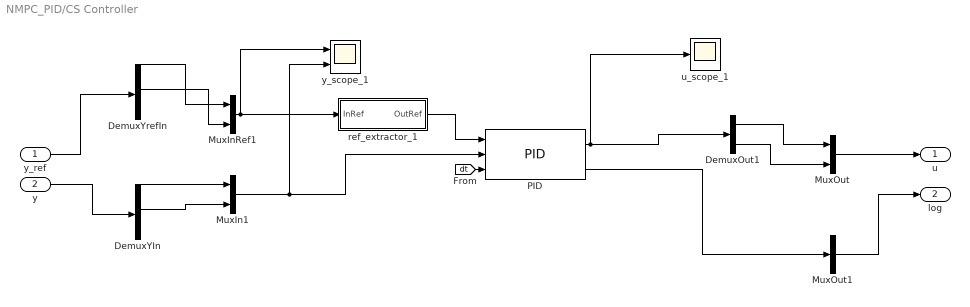
== system NMPC_PID/CS Controller ==
  y_ref : Inport  PortDimensions=12
  y : Inport  Port=2  PortDimensions=12
  DemuxOut1 : Demux  Outputs=2
  DemuxYIn : Demux  Outputs=12
  DemuxYrefIn : Demux  Outputs=12
  MuxIn1 : Mux  Inputs=2
  MuxInRef1 : Mux  Inputs=2
  MuxOut : Mux  Inputs=2
  MuxOut1 : BusCreator  Inputs=1
  PID : csbenchlab_ctl/PID  Tag=__cs_slx_ctl;__cs_comptype:ctl;__cs_compimpl:slx;  K_p=NMPC_PID_params.ctl.PID.K_p  K_i=NMPC_PID_params.ctl.PID.K_i  K_d=NMPC_PID_params.ctl.PID.K_d  K_N=NMPC_PID_params.ctl.PID.K_N  saturation_min=NMPC_PID_params.ctl.PID.saturation_min  saturation_max=NMPC_PID_params.ctl.PID.saturation_max  iid__=[56 53 56 50 101 51 101 49 45 100 101 56 53 45 52 54 54 101 45 98 52 49 50 45 52 52 97 50 54 57 99 99 100 50 98 102]  pid__=[80 73 68 58 99 115 98 101 110 99 104 108 97 98]  params=NMPC_PID_params.ctl.PID  params_struct_name=NMPC_PID_params.ctl.PID
  ref_extractor_1 : Subsystem
  u_scope_1 : Scope
  y_scope_1 : Scope  NumInputPorts=2
  u : Outport  PortDimensions=2
  log : Outport  Port=2
  wires:
  [dt] -> PID/3
  y/1 -> DemuxYIn/1
  y_ref/1 -> DemuxYrefIn/1
  MuxOut/1 -> u/1
  MuxOut1/1 -> log/1
  MuxInRef1/1 -> ref_extractor_1/1(InRef), y_scope_1/1
  ref_extractor_1/1(OutRef) -> PID/1
  MuxIn1/1 -> PID/2, y_scope_1/2
  PID/1 -> DemuxOut1/1, u_scope_1/1
  PID/2 -> MuxOut1/1
  DemuxYIn/1 -> MuxIn1/1
  DemuxYrefIn/1 -> MuxInRef1/1
  DemuxYIn/6 -> MuxIn1/2
  DemuxYrefIn/6 -> MuxInRef1/2
  DemuxOut1/1 -> MuxOut/1
  DemuxOut1/2 -> MuxOut/2

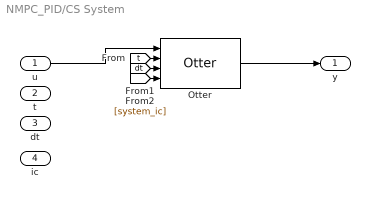
== system NMPC_PID/CS System ==
  u : Inport
  t : Inport  Port=2
  dt : Inport  Port=3
  ic : Inport  Port=4
  Otter : marine_lib_sys/Otter  Tag=system;__cs_slx_sys;__cs_comptype:sys;__cs_compimpl:slx;  payload_mass=NMPC_PID_params.sys.Otter.payload_mass  payload_location=NMPC_PID_params.sys.Otter.payload_location  current_speed=NMPC_PID_params.sys.Otter.current_speed  current_direction=NMPC_PID_params.sys.Otter.current_direction  out_gain=NMPC_PID_params.sys.Otter.out_gain  iid__=[52 97 48 100 49 48 49 48 45 52 53 52 57 45 52 100 53 49 45 98 51 97 53 45 54 48 50 101 55 99 57 51 50 98 52 53]  pid__=[79 116 116 101 114 58 109 97 114 105 110 101 95 108 105 98]  params=ActiveExperiment.SystemParams  params_struct_name=NMPC_PID_params.sys.Otter
  y : Outport
  wires:
  u/1 -> Otter/1
  Otter/1 -> y/1
  [t] -> Otter/2
  [dt] -> Otter/3
  [system_ic] -> Otter/4

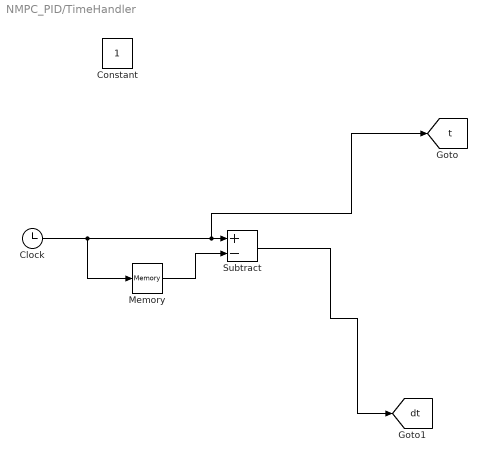
== system NMPC_PID/TimeHandler ==
  Clock : Clock
  Constant : Constant
  Memory : Memory
  Subtract : Sum  Inputs=+-
  tag scope: dt=global, t=global
  wires:
  Clock/1 -> [t], Subtract/1, Memory/1
  Memory/1 -> Subtract/2
  Subtract/1 -> [dt]

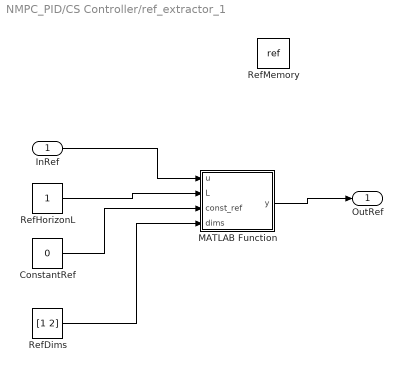
== system NMPC_PID/CS Controller/ref_extractor_1 ==
  InRef : Inport
  ConstantRef : Constant  Value=0
  MATLAB Function : MATLAB Function  TreatAsAtomicUnit=on
  RefDims : Constant  Value=[1 2]
  RefHorizonL : Constant
  RefMemory : DataStoreMemory  DataStoreName=ref  WriteAfterWriteMsg=warning  ShowAdditionalParam=off  OutDataTypeStr=double
  OutRef : Outport
  wires:
  ConstantRef/1 -> MATLAB Function/3(const_ref)
  RefDims/1 -> MATLAB Function/4(dims)
  RefHorizonL/1 -> MATLAB Function/2(L)
  InRef/1 -> MATLAB Function/1(u)
  MATLAB Function/1(y) -> OutRef/1

== matlab function NMPC_PID/MATLAB Function ==
  settings: updateMethod=DISCRETE
  data: waypoints input; vel input; pose input; u output; params parameter; reference_path output
function [u, reference_path] = fcn(waypoints, vel, pose, params)

    persistent global_path idx initial_global_path
    use_waypoints = 0;
    num_divs = 100;        
    if isempty(global_path)

        if use_waypoints
            global_path = zeros((height(waypoints)-1) * num_divs+1, 3);
            global_path(1, :) = waypoints(1, :);
            for i=1:length(waypoints)-1
                global_path(2 + (i-1)*num_divs : i*num_divs+1, :) = get_traj_between(waypoints(i, :), waypoints(i+1, :), num_divs);
            end
            idx = 1;
        else
            global_path = zeros((height(waypoints)-1) * num_divs+1, 3);
            global_path(1, :) = waypoints(1, :);
            k=5;
            kx=1.3;
            ky=0;
            L = 200;
            N = 5;
            theta=linspace(0, 2*N*pi, L);
            r = k*theta;
            x = k*(cos(theta)-1) + kx*theta;
            y = k*sin(theta) + ky*theta;
            global_path(2:L+1, :) = [x' y' zeros(L, 1)] + repmat(global_path(1, :), L, 1);
            global_path(L+2:end, :) = repmat(global_path(L+1, :), length(global_path) - L-1, 1);
            idx = 1;
        end
        initial_global_path = global_path;
    end
    reference_path = initial_global_path;
    L = 10;
    u = zeros(L, 12);
    coder.extrinsic('kinematic_nmpc');
    u_res = kinematic_nmpc(global_path, pose, vel, L, params);
    u(:, 1) = u_res(1:L, 1);
    u(:, 6) = u_res(1:L, 2);
end

== matlab function NMPC_PID/CS Controller/ref_extractor_1/MATLAB Function ==
  settings: updateMethod=DISCRETE
  data: u input; L input; const_ref input; dims input; y output; ref data_store_memory; GlobalReference parameter
function y = fcn(u, L, const_ref, dims, GlobalReference)

persistent cnt
global ref

if isempty(cnt)
    cnt = 0;
end

if GlobalReference == 0
    y = repmat(u', 1);
    return;
end


cnt = cnt+1;

horizon_end = cnt+L-1;
if L > 1 
   if horizon_end > length(GlobalReference)
        if size(ref, 1) == size(u, 1)
            y = permute(ref, [2, 1]);
        else
            y = ref;
        end       
        return
   end

   if size(ref, 1) == size(u, 1)
      
      if const_ref == 0
        ref(:, :) = GlobalReference(cnt:horizon_end, dims)';
      else
        ref(:, :) = repmat(GlobalReference(cnt, dims)', 1, L);
      end
      y = permute(ref, [2, 1]);
   else
      if const_ref == 0
        ref(1:L, :) = GlobalReference(cnt:horizon_end, dims);
      else
        ref(1:L, :) = repmat(GlobalReference(cnt, dims), L, 1);
      end
      y = ref;
   end
else
   if size(ref, 1) == size(u, 1)
       ref = u;
       y = permute(ref, [2, 1]);
   else
      ref(1, :) = u';
      y = ref;
   end
end
